simulink model "asmathew_adaptive_control"  (R2021a)
settings: Solver=VariableStepAuto  StartTime=0.0  StopTime=10.0  RelTol=1e-3
settings Model: Creator=Aaron  LastModifiedBy=Aaron

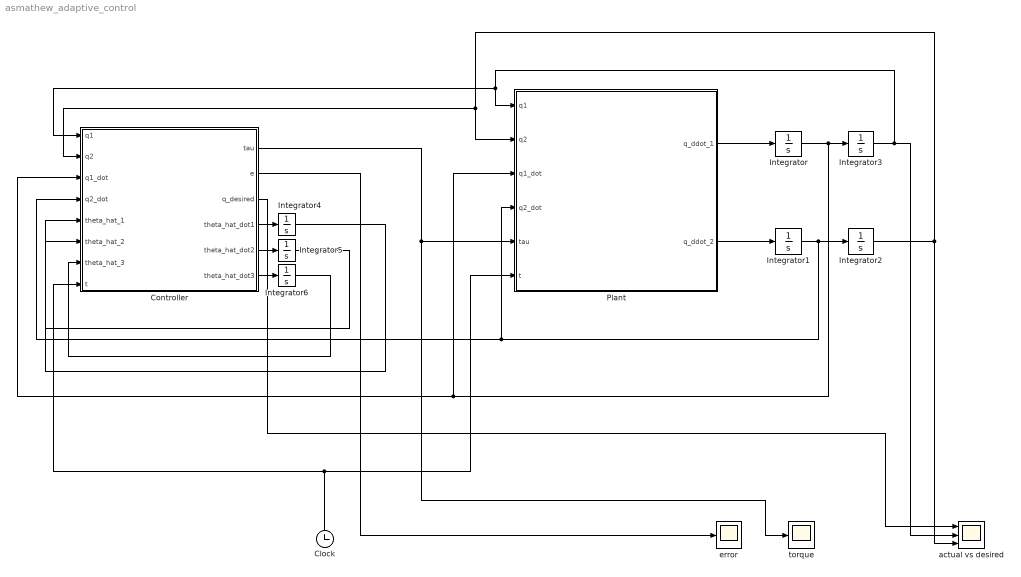
== system asmathew_adaptive_control ==
  Clock : Clock
  Controller : MATLAB Function  TreatAsAtomicUnit=on
  Integrator{,1..6} (7 alike) : Integrator
  Plant : MATLAB Function  TreatAsAtomicUnit=on
  actual vs desired : Scope  NumInputPorts=3
  error : Scope
  torque : Scope
  wires:
  Plant/1(q_ddot_1) -> Integrator/1
  Plant/2(q_ddot_2) -> Integrator1/1
  Integrator1/1 -> Plant/4(q2_dot), Controller/4(q2_dot), Integrator2/1
  Integrator/1 -> Plant/3(q1_dot), Controller/3(q1_dot), Integrator3/1
  Integrator3/1 -> actual vs desired/2, Controller/1(q1), Plant/1(q1)
  Integrator2/1 -> Plant/2(q2), Controller/2(q2), actual vs desired/3
  Controller/1(tau) -> Plant/5(tau), torque/1
  Clock/1 -> Plant/6(t), Controller/8(t)
  Controller/4(theta_hat_dot1) -> Integrator4/1
  Controller/5(theta_hat_dot2) -> Integrator5/1
  Controller/6(theta_hat_dot3) -> Integrator6/1
  Integrator4/1 -> Controller/5(theta_hat_1)
  Integrator5/1 -> Controller/6(theta_hat_2)
  Integrator6/1 -> Controller/7(theta_hat_3)
  Controller/2(e) -> error/1
  Controller/3(q_desired) -> actual vs desired/1

== matlab function asmathew_adaptive_control/Controller ==
  data: q1 input; tau output; e output; q_desired output; q2 input; q1_dot input; q2_dot input; theta_hat_1 input; theta_hat_2 input; theta_hat_3 input; t input; theta_hat_dot1 output; theta_hat_dot2 output; theta_hat_dot3 output
function [tau,e,q_desired,theta_hat_dot1,theta_hat_dot2,theta_hat_dot3] = fcn(q1,q2,q1_dot,q2_dot,theta_hat_1,theta_hat_2,theta_hat_3,t)

% initialzing given constants p1,p2,p3,fd1,fd2
% p1,p2,p3 have units Kg.m^2
% fd1 and fd2 have units Nm.sec

p1 = 3.473;
p2 = 0.196;
p3 = 0.242;

fd1 = 5.3;
fd2 = 1.1;

alpha = 150;
k = 85;
gamma = 2;

F = [fd1 0 ; 0 fd2];
% Compute M , Vm
M = [p1+2*p3*cos(q2) p2+p3*cos(q2); p2+p3*cos(q2) p2];
Vm = [-p3*sin(q2)*q2_dot -p3*sin(q2)*(q2_dot+q1_dot); p3*sin(q2)*q1_dot 0];

% Define a desired signal

qd1 = 3*sin(5*pi*t);
qd2 = 6*sin(2*t);

qd1_dot = 15*pi*cos(5*t);
qd2_dot = 12*cos(2*t);

qd1_ddot = -75*pi^2*sin(5*pi*t);
qd2_ddot = -24*sin(2*t);

q_desired = [qd1;qd2];
q_actual = [q1;q2];


qd_dot = [qd1_dot;qd2_dot];
q_actual_dot = [q1_dot;q2_dot];

qd_ddot = [qd1_ddot;qd2_ddot];

% Obtain the tracking signal
e = q_desired - q_actual;
e_dot = q_desired - q_actual_dot;

% Define an auxilary signal
r = e_dot + (alpha*e);

% Code for Adaptive Controller
Y = [qd_ddot+alpha*e alpha*e+qd_dot q_actual_dot];
theta = [M; Vm; F];
theta_hat_dot = inv(gamma)* Y' *r ;
theta_hat_dot1 = theta_hat_dot(1);
theta_hat_dot2 = theta_hat_dot(2);
theta_hat_dot3 = theta_hat_dot(3);
theta_hat = [theta_hat_1;theta_hat_2;theta_hat_3];
tau = k*r + Y*theta_hat;

== matlab function asmathew_adaptive_control/Plant ==
  data: q1 input; q2 input; q1_dot input; q2_dot input; q_ddot_1 output; q_ddot_2 output; tau input; t input
function [q_ddot_1,q_ddot_2]= fcn(q1,q2,q1_dot,q2_dot,tau,t)

% initialzing given constants p1,p2,p3,fd1,fd2
% p1,p2,p3 have units Kg.m^2
% fd1 and fd2 have units Nm.sec

p1 = 3.473;
p2 = 0.196;
p3 = 0.242;

fd1 = 5.3;
fd2 = 1.1;

% Compute M , Vm
M = [p1+2*p3*cos(q2) p2+p3*cos(q2); p2+p3*cos(q2) p2];
Vm = [-p3*sin(q2)*q2_dot -p3*sin(q2)*(q2_dot+q1_dot); p3*sin(q2)*q1_dot 0];

% Initialize F matrix
F = [fd1 0 ; 0 fd2];

%%q_ddot should be a 2 x 1 matrix
q_dot_matrix = [q1_dot; q2_dot];

%% inv(M) * ((-Vm * q_dot_matrix) - (F*q_dot_matrix))

% Add disturbance term t_dist 
q_ddot = inv(M)*((-Vm * q_dot_matrix) - (F*q_dot_matrix) + tau);

q_ddot_1 = q_ddot(1);
q_ddot_2 = q_ddot(2);
